simulink model "FOC_2020b"  (R2021a)
settings: Solver=ode23t  StartTime=0.0  StopTime=0.1  RelTol=1e-3  AbsTol=1e-3  EnableMultiTasking=on
values from neighbouring files (symbols this model uses):
  f_c = 10000    [FOC_params.m]
  Kpd = Ld*2*pi*BW    (= 0.0753982236862)    [FOC_params.m]
  Kpn = Kpq/(Lq*d*K)    (= 1.22461076833)    [FOC_params.m]
  Kpq = Lq*2*pi*BW    (= 0.125663706144)    [FOC_params.m]
  Kr = 270    [FOC_params.m]
  Ld = 0.00003    (= 3e-05)    [FOC_params.m]
  Lq = 0.00005    (= 5e-05)    [FOC_params.m]
  np = 5    [FOC_params.m]
  PERIOD = 3750    [FOC_params.m]
  psiPM = 0.007    [FOC_params.m]
  R = 0.023    [FOC_params.m]
  T_dead = 2.0e-6    (= 2e-06)    [FOC_params.m]
  Tnd = Ld/R    (= 0.00130434782609)    [FOC_params.m]
  Tnn = d^2*Lq/Kpq    (= 0.039788735773)    [FOC_params.m]
  Tnq = Lq/R    (= 0.00217391304348)    [FOC_params.m]
  u_dc = 12    [FOC_params.m]
libraries: nesl_utility x23, ee_lib x22, fl_lib x22, pid_lib x3, simulink x3, cstblocks x2, spsAlphaBetaZerotodq0Lib x1, spsabctoAlphaBetaZeroLib x1, spsdq0toAlphaBetaZeroLib x1, spsTriangleGeneratorLib x1
(part 2 of 2)

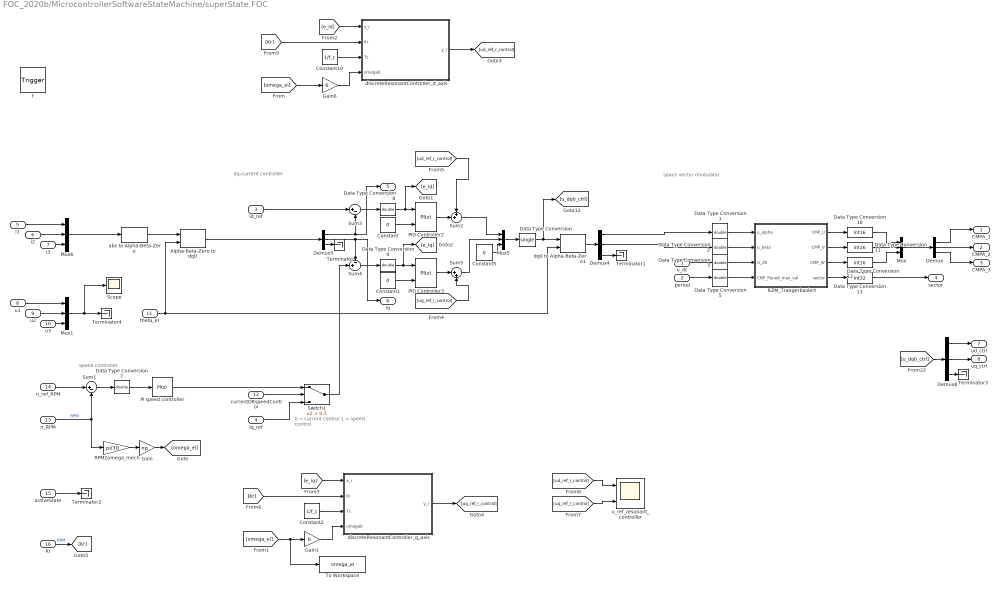
== system FOC_2020b/MicrocontrollerSoftwareStateMachine/superState.FOC ==
  note: speed controller
  note: space vector modulator
  note: dq-current controller
  note: 0 = current control
      | 1 = speed control
  u_dc : Inport  OutDataTypeStr=single  PortDimensions=1
  period : Inport  Port=2  OutDataTypeStr=uint16  PortDimensions=1
  id_ref : Inport  Port=3  OutDataTypeStr=single  PortDimensions=1
  iq_ref : Inport  Port=4  OutDataTypeStr=single  PortDimensions=1
  i1 : Inport  Port=5  OutDataTypeStr=single  PortDimensions=1
  i2 : Inport  Port=6  OutDataTypeStr=single  PortDimensions=1
  i3 : Inport  Port=7  OutDataTypeStr=single  PortDimensions=1
  u1 : Inport  Port=8  OutDataTypeStr=single  PortDimensions=1
  u2 : Inport  Port=9  OutDataTypeStr=single  PortDimensions=1
  u3 : Inport  Port=10  OutDataTypeStr=single  PortDimensions=1
  theta_el : Inport  Port=11  OutDataTypeStr=single  PortDimensions=1
  currentORspeedControl : Inport  Port=12  OutDataTypeStr=boolean  PortDimensions=1
  n_RPM : Inport  Port=13  OutDataTypeStr=single  PortDimensions=1
  n_ref_RPM : Inport  Port=14  OutDataTypeStr=single  PortDimensions=1
  activeState : Inport  Port=15  OutDataTypeStr=uint8  PortDimensions=1
  Kr : Inport  Port=16  OutDataTypeStr=single  PortDimensions=1
  f : TriggerPort  TriggerType=function-call  VariantControl=(inherit)
      settings: CopyFcn=Stateflow.SLINSF.SimulinkMan.removeBlockPreDeleteFcn  PreDeleteFcn=Stateflow.SLINSF.SimulinkMan.unsafePredeleteFcn
  Alpha-Beta-Zero to dq0 : spsAlphaBetaZerotodq0Lib/Alpha-Beta-Zero to dq0  Alignment=Aligned with phase A axis
      settings: SourceProductBaseCode=PS
  Constant : Constant  Value=0
  Constant1 : Constant  Value=0
  Constant10 : Constant  Value=1/f_c
  Constant2 : Constant  Value=1/f_c
  Constant5 : Constant  Value=0
  Data Type Conversion : DataTypeConversion  OutDataTypeStr=single
  Data Type Conversion{1..3,5,7..9} (7 alike) : DataTypeConversion  OutDataTypeStr=double
  Data Type Conversion10 : DataTypeConversion  OutDataTypeStr=int16
  Data Type Conversion11 : DataTypeConversion  OutDataTypeStr=int16
  Data Type Conversion12 : DataTypeConversion  OutDataTypeStr=int16
  Data Type Conversion13 : DataTypeConversion  OutDataTypeStr=int32
  Demux{,4..5,8} (4 alike) : Demux  Outputs=3
  Gain : Gain  Gain=np
  Gain1 : Gain  Gain=6
  Gain6 : Gain  Gain=6
  Mux{,1,5..6} (4 alike) : Mux  Inputs=3
  PI speed controller : pid_lib/PID Controller  Controller=PI  Form=Ideal  TimeDomain=Discrete-time  UseExternalTs=off  SampleTime=-1  IntegratorMethod=Forward Euler  FilterMethod=Forward Euler  ControllerParametersSource=internal  P=Kpn  I=1/Tnn  D=0  UseFilter=on  N=100  TunerSelectOption=Transfer Function Based (PID Tuner App)  InitialConditionSource=internal  InitialConditionForIntegrator=0  InitialConditionForFilter=0  DifferentiatorICPrevScaledInput=0  ExternalReset=none  TrackingMode=off  Kt=1  LimitOutput=on  SatLimitsSource=internal  UpperSaturationLimit=10  LowerSaturationLimit=-10  LinearizeAsGain=on  AntiWindupMode=clamping  Kb=1  POutMin=[]  POutMax=[]  IOutMin=[]  IOutMax=[]  DOutMin=[]  DOutMax=[]  NOutMin=[]  NOutMax=[]  SumOutMin=[]  SumOutMax=[]  SaturationOutMin=[]  SaturationOutMax=[]  PParamMin=[]  PParamMax=[]  IParamMin=[]  IParamMax=[]  DParamMin=[]  DParamMax=[]  NParamMin=[]  NParamMax=[]  KbParamMin=[]  KbParamMax=[]  KtParamMin=[]  KtParamMax=[]  KbOutMin=[]  KbOutMax=[]  KtOutMin=[]  KtOutMax=[]  IntegratorOutMin=[]  IntegratorOutMax=[]  FilterOutMin=[]  FilterOutMax=[]  SumI1OutMin=[]  SumI1OutMax=[]  SumI2OutMin=[]  SumI2OutMax=[]  SumI3OutMin=[]  SumI3OutMax=[]  SumI4OutMin=[]  SumI4OutMax=[]  SumDOutMin=[]  SumDOutMax=[]  DifferentiatorOutMin=[]  DifferentiatorOutMax=[]  FilterDiffOutCoefMin=[]  FilterDiffOutCoefMax=[]  ReciprocalOutMin=[]  ReciprocalOutMax=[]  SumDenOutMin=[]  SumDenOutMax=[]  SumNumOutMin=[]  SumNumOutMax=[]  DivideOutMin=[]  DivideOutMax=[]  UdiffTsProdOutMin=[]  UdiffTsProdOutMax=[]  NTsProdOutMin=[]  NTsProdOutMax=[]  UintegralTsProdOutMin=[]  UintegralTsProdOutMax=[]  UngainTsProdOutMin=[]  UngainTsProdOutMax=[]  IntegratorContinuousStateAttributes=''  IntegratorStateMustResolveToSignalObject=off  IntegratorRTWStateStorageClass=Auto  FilterContinuousStateAttributes=''  FilterStateMustResolveToSignalObject=off  FilterRTWStateStorageClass=Auto  ParallelPVariant=Passthrough  IdealPVariant=InternalParameters  IVariant=InternalParameters  DVariant=Disabled  IntegratorVariant=Discrete  SatVariant=Enabled  AWVariant=DiscClampingIdeal  PCopyVariant=InternalParamsIdeal  TRVariant=Disabled  FdbkBlocksVariant=Forward  IdealPFdbkVariant=Disabled  SatFdbkVariant=Disabled  DerivativeFilterVariant=Disabled  NVariant=Disabled  NCopyVariant=Disabled_SignalSpec  FilterICVariant=Disabled  IntegratorICVariant=InternalICs  ExternalResetVariant=Disabled  TRSumVariant=Passthrough  SumFdbkVariant=Disabled  SumVariant=Sum_PI  TsampFilterVariant=InternalTs  TsampNgainVariant=Passthrough  TsampIntegralVariant=Passthrough  ExternalSaturationOutDataTypeStr=Inherit: Same as second input
  PID Controller2 : pid_lib/PID Controller  Controller=PI  Form=Ideal  TimeDomain=Discrete-time  UseExternalTs=off  SampleTime=-1  IntegratorMethod=Forward Euler  FilterMethod=Forward Euler  ControllerParametersSource=internal  P=Kpd  I=1/Tnd  D=0  UseFilter=on  N=100  TunerSelectOption=Transfer Function Based (PID Tuner App)  InitialConditionSource=internal  InitialConditionForIntegrator=0  InitialConditionForFilter=0  DifferentiatorICPrevScaledInput=0  ExternalReset=rising  TrackingMode=off  Kt=1  LimitOutput=on  SatLimitsSource=internal  UpperSaturationLimit=12  LowerSaturationLimit=-12  LinearizeAsGain=on  AntiWindupMode=clamping  Kb=1  POutMin=[]  POutMax=[]  IOutMin=[]  IOutMax=[]  DOutMin=[]  DOutMax=[]  NOutMin=[]  NOutMax=[]  SumOutMin=[]  SumOutMax=[]  SaturationOutMin=[]  SaturationOutMax=[]  PParamMin=[]  PParamMax=[]  IParamMin=[]  IParamMax=[]  DParamMin=[]  DParamMax=[]  NParamMin=[]  NParamMax=[]  KbParamMin=[]  KbParamMax=[]  KtParamMin=[]  KtParamMax=[]  KbOutMin=[]  KbOutMax=[]  KtOutMin=[]  KtOutMax=[]  IntegratorOutMin=[]  IntegratorOutMax=[]  FilterOutMin=[]  FilterOutMax=[]  SumI1OutMin=[]  SumI1OutMax=[]  SumI2OutMin=[]  SumI2OutMax=[]  SumI3OutMin=[]  SumI3OutMax=[]  SumI4OutMin=[]  SumI4OutMax=[]  SumDOutMin=[]  SumDOutMax=[]  DifferentiatorOutMin=[]  DifferentiatorOutMax=[]  FilterDiffOutCoefMin=[]  FilterDiffOutCoefMax=[]  ReciprocalOutMin=[]  ReciprocalOutMax=[]  SumDenOutMin=[]  SumDenOutMax=[]  SumNumOutMin=[]  SumNumOutMax=[]  DivideOutMin=[]  DivideOutMax=[]  UdiffTsProdOutMin=[]  UdiffTsProdOutMax=[]  NTsProdOutMin=[]  NTsProdOutMax=[]  UintegralTsProdOutMin=[]  UintegralTsProdOutMax=[]  UngainTsProdOutMin=[]  UngainTsProdOutMax=[]  IntegratorContinuousStateAttributes=''  IntegratorStateMustResolveToSignalObject=off  IntegratorRTWStateStorageClass=Auto  FilterContinuousStateAttributes=''  FilterStateMustResolveToSignalObject=off  FilterRTWStateStorageClass=Auto  ParallelPVariant=Passthrough  IdealPVariant=InternalParameters  IVariant=InternalParameters  DVariant=Disabled  IntegratorVariant=Discrete  SatVariant=Enabled  AWVariant=DiscClampingIdeal  PCopyVariant=InternalParamsIdeal  TRVariant=Disabled  FdbkBlocksVariant=Forward  IdealPFdbkVariant=Disabled  SatFdbkVariant=Disabled  DerivativeFilterVariant=Disabled  NVariant=Disabled  NCopyVariant=Disabled_SignalSpec  FilterICVariant=Disabled  IntegratorICVariant=InternalICs  ExternalResetVariant=ExternalReset  TRSumVariant=Passthrough  SumFdbkVariant=Disabled  SumVariant=Sum_PI  TsampFilterVariant=InternalTs  TsampNgainVariant=Passthrough  TsampIntegralVariant=Passthrough  ExternalSaturationOutDataTypeStr=Inherit: Same as second input
  PID Controller3 : pid_lib/PID Controller  Controller=PI  Form=Ideal  TimeDomain=Discrete-time  UseExternalTs=off  SampleTime=-1  IntegratorMethod=Forward Euler  FilterMethod=Forward Euler  ControllerParametersSource=internal  P=Kpq  I=1/Tnq  D=0  UseFilter=on  N=100  TunerSelectOption=Transfer Function Based (PID Tuner App)  InitialConditionSource=internal  InitialConditionForIntegrator=0  InitialConditionForFilter=0  DifferentiatorICPrevScaledInput=0  ExternalReset=rising  TrackingMode=off  Kt=1  LimitOutput=on  SatLimitsSource=internal  UpperSaturationLimit=12  LowerSaturationLimit=-12  LinearizeAsGain=on  AntiWindupMode=clamping  Kb=1  POutMin=[]  POutMax=[]  IOutMin=[]  IOutMax=[]  DOutMin=[]  DOutMax=[]  NOutMin=[]  NOutMax=[]  SumOutMin=[]  SumOutMax=[]  SaturationOutMin=[]  SaturationOutMax=[]  PParamMin=[]  PParamMax=[]  IParamMin=[]  IParamMax=[]  DParamMin=[]  DParamMax=[]  NParamMin=[]  NParamMax=[]  KbParamMin=[]  KbParamMax=[]  KtParamMin=[]  KtParamMax=[]  KbOutMin=[]  KbOutMax=[]  KtOutMin=[]  KtOutMax=[]  IntegratorOutMin=[]  IntegratorOutMax=[]  FilterOutMin=[]  FilterOutMax=[]  SumI1OutMin=[]  SumI1OutMax=[]  SumI2OutMin=[]  SumI2OutMax=[]  SumI3OutMin=[]  SumI3OutMax=[]  SumI4OutMin=[]  SumI4OutMax=[]  SumDOutMin=[]  SumDOutMax=[]  DifferentiatorOutMin=[]  DifferentiatorOutMax=[]  FilterDiffOutCoefMin=[]  FilterDiffOutCoefMax=[]  ReciprocalOutMin=[]  ReciprocalOutMax=[]  SumDenOutMin=[]  SumDenOutMax=[]  SumNumOutMin=[]  SumNumOutMax=[]  DivideOutMin=[]  DivideOutMax=[]  UdiffTsProdOutMin=[]  UdiffTsProdOutMax=[]  NTsProdOutMin=[]  NTsProdOutMax=[]  UintegralTsProdOutMin=[]  UintegralTsProdOutMax=[]  UngainTsProdOutMin=[]  UngainTsProdOutMax=[]  IntegratorContinuousStateAttributes=''  IntegratorStateMustResolveToSignalObject=off  IntegratorRTWStateStorageClass=Auto  FilterContinuousStateAttributes=''  FilterStateMustResolveToSignalObject=off  FilterRTWStateStorageClass=Auto  ParallelPVariant=Passthrough  IdealPVariant=InternalParameters  IVariant=InternalParameters  DVariant=Disabled  IntegratorVariant=Discrete  SatVariant=Enabled  AWVariant=DiscClampingIdeal  PCopyVariant=InternalParamsIdeal  TRVariant=Disabled  FdbkBlocksVariant=Forward  IdealPFdbkVariant=Disabled  SatFdbkVariant=Disabled  DerivativeFilterVariant=Disabled  NVariant=Disabled  NCopyVariant=Disabled_SignalSpec  FilterICVariant=Disabled  IntegratorICVariant=InternalICs  ExternalResetVariant=ExternalReset  TRSumVariant=Passthrough  SumFdbkVariant=Disabled  SumVariant=Sum_PI  TsampFilterVariant=InternalTs  TsampNgainVariant=Passthrough  TsampIntegralVariant=Passthrough  ExternalSaturationOutDataTypeStr=Inherit: Same as second input
  RPM2omega_mech : Gain  Gain=pi/30
  RZM_Traegerbasiert : MATLAB Function  TreatAsAtomicUnit=on
  Scope : Scope
  Sum1 : Sum  Inputs=|+-
  Sum2 : Sum  Inputs=++|
  Sum3 : Sum  Inputs=|+-
  Sum4 : Sum  Inputs=-+|
  Sum5 : Sum  Inputs=|++
  Switch1 : Switch  Criteria=u2 > Threshold  Threshold=0.5
  Terminator{,1..4} (5 alike) : Terminator
  To Workspace : ToWorkspace  VariableName=omega_el  SaveFormat=Timeseries  SampleTime=-1
  abc to Alpha-Beta-Zero : spsabctoAlphaBetaZeroLib/abc to Alpha-Beta-Zero
      settings: SourceProductBaseCode=PS
  discreteResonantController_d_axis : Subsystem
  discreteResonantController_q_axis : Subsystem
  dq0 to Alpha-Beta-Zero1 : spsdq0toAlphaBetaZeroLib/dq0 to Alpha-Beta-Zero  Alignment=Aligned with phase A axis
      settings: SourceProductBaseCode=PS
  u_ref_resonant_controller : Scope  NumInputPorts=2
  CMPA_1 : Outport  OutDataTypeStr=int16  PortDimensions=1  VectorParamsAs1DForOutWhenUnconnected=off
  CMPA_2 : Outport  Port=2  OutDataTypeStr=int16  PortDimensions=1  VectorParamsAs1DForOutWhenUnconnected=off
  CMPA_3 : Outport  Port=3  OutDataTypeStr=int16  PortDimensions=1  VectorParamsAs1DForOutWhenUnconnected=off
  sector : Outport  Port=4  OutDataTypeStr=int32  PortDimensions=1  VectorParamsAs1DForOutWhenUnconnected=off
  id : Outport  Port=5  OutDataTypeStr=single  PortDimensions=1  VectorParamsAs1DForOutWhenUnconnected=off
  iq : Outport  Port=6  OutDataTypeStr=single  PortDimensions=1  VectorParamsAs1DForOutWhenUnconnected=off
  ud_ctrl : Outport  Port=7  OutDataTypeStr=single  PortDimensions=1  VectorParamsAs1DForOutWhenUnconnected=off
  uq_ctrl : Outport  Port=8  OutDataTypeStr=single  PortDimensions=1  VectorParamsAs1DForOutWhenUnconnected=off
  wires:
  i2/1 -> Mux6/2
  Demux4/3 -> Terminator1/1
  RZM_Traegerbasiert/1(CMP_U) -> Data Type Conversion10/1
  Constant5/1 -> Mux5/3
  dq0 to Alpha-Beta-Zero1/1 -> Demux4/1
  Demux5/2 -> iq/1, Sum4/1
  Demux5/3 -> Terminator/1
  Sum3/1 -> Data Type Conversion8/1
  Data Type Conversion1/1 -> RZM_Traegerbasiert/1(u_alpha)
  i3/1 -> Mux6/3
  Demux5/1 -> id/1, Sum3/2
  Data Type Conversion2/1 -> RZM_Traegerbasiert/2(u_beta)
  Alpha-Beta-Zero to dq0/1 -> Demux5/1
  Mux5/1 -> Data Type Conversion/1
  RZM_Traegerbasiert/3(CMP_W) -> Data Type Conversion12/1
  Switch1/1 -> Sum4/2
  Sum4/1 -> Data Type Conversion9/1
  u_dc/1 -> Data Type Conversion3/1
  RZM_Traegerbasiert/2(CMP_V) -> Data Type Conversion11/1
  RZM_Traegerbasiert/4(sector) -> Data Type Conversion13/1
  Data Type Conversion3/1 -> RZM_Traegerbasiert/3(U_ZK)
  id_ref/1 -> Sum3/1
  Data Type Conversion5/1 -> RZM_Traegerbasiert/4(CMP_Period_max_val)
  Data Type Conversion/1 -> [u_dq0_ctrl], dq0 to Alpha-Beta-Zero1/1
  Data Type Conversion8/1 -> [e_id], PID Controller2/1
  Data Type Conversion9/1 -> [e_iq], PID Controller3/1
  Demux4/1 -> Data Type Conversion1/1
  Demux4/2 -> Data Type Conversion2/1
  period/1 -> Data Type Conversion5/1
  Data Type Conversion11/1 -> Mux/2
  Data Type Conversion10/1 -> Mux/1
  Data Type Conversion12/1 -> Mux/3
  Mux/1 -> Demux/1
  Data Type Conversion13/1 -> sector/1
  i1/1 -> Mux6/1
  u1/1 -> Mux1/1
  u2/1 -> Mux1/2
  u3/1 -> Mux1/3
  Mux6/1 -> abc to Alpha-Beta-Zero/1
  abc to Alpha-Beta-Zero/1 -> Alpha-Beta-Zero to dq0/1
  Mux1/1 -> Scope/1, Terminator4/1
  theta_el/1 -> dq0 to Alpha-Beta-Zero1/2, Alpha-Beta-Zero to dq0/2
  iq_ref/1 -> Switch1/3
  currentORspeedControl/1 -> Switch1/2
  Data Type Conversion7/1 -> PI speed controller/1
  PI speed controller/1 -> Switch1/1
  Sum1/1 -> Data Type Conversion7/1
  n_ref_RPM/1 -> Sum1/1
  Constant1/1 -> PID Controller3/2
  Constant/1 -> PID Controller2/2
  activeState/1 -> Terminator2/1
  [u_dq0_ctrl] -> Demux8/1
  Demux8/3 -> Terminator3/1
  Demux8/2 -> uq_ctrl/1
  Demux8/1 -> ud_ctrl/1
  Demux/1 -> CMPA_1/1
  Demux/3 -> CMPA_3/1
  Demux/2 -> CMPA_2/1
  PID Controller2/1 -> Sum2/2
  PID Controller3/1 -> Sum5/1
  n_RPM/1 -> RPM2omega_mech/1, Sum1/2  "RPM"
  Gain6/1 -> discreteResonantController_d_axis/4(omega0)
  [Kr] -> discreteResonantController_d_axis/2(Kr)
  [omega_el] -> Gain6/1
  [e_id] -> discreteResonantController_d_axis/1(x_r)
  Constant10/1 -> discreteResonantController_d_axis/3(Ts)
  discreteResonantController_d_axis/1(y_r) -> [ud_ref_r_control]
  [omega_el] -> To Workspace/1, Gain1/1
  discreteResonantController_q_axis/1(y_r) -> [uq_ref_r_control]
  [e_iq] -> discreteResonantController_q_axis/1(x_r)
  Constant2/1 -> discreteResonantController_q_axis/3(Ts)
  Gain1/1 -> discreteResonantController_q_axis/4(omega0)
  Sum2/1 -> Mux5/1
  Sum5/1 -> Mux5/2
  RPM2omega_mech/1 -> Gain/1
  Gain/1 -> [omega_el]
  [uq_ref_r_control] -> Sum5/2
  [ud_ref_r_control] -> Sum2/1
  [Kr] -> discreteResonantController_q_axis/2(Kr)
  Kr/1 -> [Kr]  "RPM"
  [uq_ref_r_control] -> u_ref_resonant_controller/2
  [ud_ref_r_control] -> u_ref_resonant_controller/1

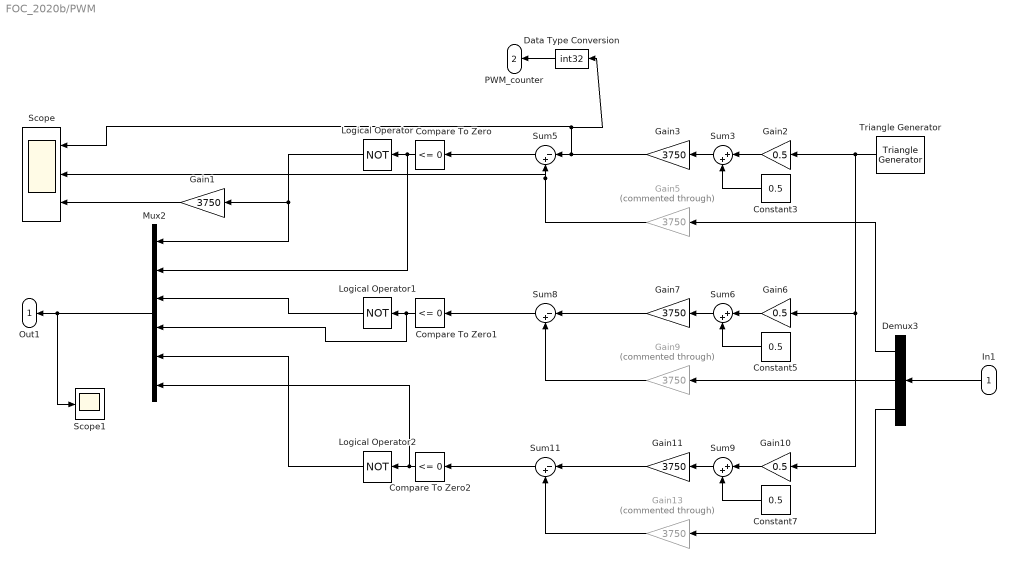
== system FOC_2020b/PWM ==
  In1 : Inport
  Compare To Zero : simulink/Logic and Bit Operations/Compare To Zero  relop=<=  OutDataTypeStr=boolean
  Compare To Zero1 : simulink/Logic and Bit Operations/Compare To Zero  relop=<=  OutDataTypeStr=boolean
  Compare To Zero2 : simulink/Logic and Bit Operations/Compare To Zero  relop=<=  OutDataTypeStr=boolean
  Constant3 : Constant  Value=0.5
  Constant5 : Constant  Value=0.5
  Constant7 : Constant  Value=0.5
  Data Type Conversion : DataTypeConversion  OutDataTypeStr=int32
  Demux3 : Demux  Outputs=3
  Gain{1,3,7,11} (4 alike) : Gain  Gain=3750  ParamDataTypeStr=single
  Gain10 : Gain  Gain=0.5
  Gain13 : Gain  Commented=through  Gain=3750  ParamDataTypeStr=single
  Gain2 : Gain  Gain=0.5
  Gain5 : Gain  Commented=through  Gain=3750  ParamDataTypeStr=single
  Gain6 : Gain  Gain=0.5
  Gain9 : Gain  Commented=through  Gain=3750  ParamDataTypeStr=single
  Logical Operator : Logic  Operator=NOT  AllPortsSameDT=off  OutDataTypeStr=boolean
  Logical Operator1 : Logic  Operator=NOT  AllPortsSameDT=off  OutDataTypeStr=boolean
  Logical Operator2 : Logic  Operator=NOT  AllPortsSameDT=off  OutDataTypeStr=boolean
  Mux2 : Mux  Inputs=6
  Scope : Scope  NumInputPorts=3
  Scope1 : Scope
  Sum11 : Sum  Inputs=|-+
  Sum3 : Sum  Inputs=|++
  Sum5 : Sum  Inputs=|-+
  Sum6 : Sum  Inputs=|++
  Sum8 : Sum  Inputs=|-+
  Sum9 : Sum  Inputs=|++
  Triangle Generator : spsTriangleGeneratorLib/Triangle Generator  Freq=20000  Phase=0  Ts=0
  Out1 : Outport  VectorParamsAs1DForOutWhenUnconnected=off
  PWM_counter : Outport  Port=2  VectorParamsAs1DForOutWhenUnconnected=off
  wires:
  Demux3/3 -> Gain13/1
  Logical Operator2/1 -> Mux2/5
  Logical Operator1/1 -> Mux2/3
  Mux2/1 -> Scope1/1, Out1/1
  Compare To Zero2/1 -> Mux2/6, Logical Operator2/1
  Gain10/1 -> Sum9/1
  Sum8/1 -> Compare To Zero1/1
  Gain6/1 -> Sum6/1
  Sum9/1 -> Gain11/1
  Triangle Generator/1 -> Gain10/1, Gain6/1, Gain2/1
  Sum6/1 -> Gain7/1
  Demux3/2 -> Gain9/1
  Compare To Zero1/1 -> Mux2/4, Logical Operator1/1
  Constant5/1 -> Sum6/2
  Constant7/1 -> Sum9/2
  Sum11/1 -> Compare To Zero2/1
  Sum3/1 -> Gain3/1
  Constant3/1 -> Sum3/2
  Demux3/1 -> Gain5/1
  Sum5/1 -> Compare To Zero/1
  Gain2/1 -> Sum3/1
  In1/1 -> Demux3/1
  Gain5/1 -> Scope/2, Sum5/2
  Gain9/1 -> Sum8/2
  Gain13/1 -> Sum11/2
  Gain3/1 -> Data Type Conversion/1, Scope/1, Sum5/1
  Gain7/1 -> Sum8/1
  Gain11/1 -> Sum11/1
  Logical Operator/1 -> Gain1/1, Mux2/1
  Compare To Zero/1 -> Mux2/2, Logical Operator/1
  Gain1/1 -> Scope/3
  Data Type Conversion/1 -> PWM_counter/1

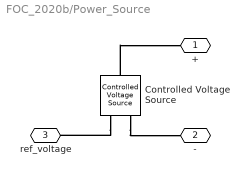
== system FOC_2020b/Power_Source ==
  Controlled Voltage Source : fl_lib/Electrical/Electrical Sources/Controlled Voltage Source
  + : PMIOPort  Side=Right
  - : PMIOPort  Port=2  Side=Right
  ref_voltage : PMIOPort  Port=3  Side=Left
  connections:
  Controlled Voltage Source/LConn1 -- +/RConn1
  Controlled Voltage Source/RConn2 -- -/RConn1
  Controlled Voltage Source/RConn1 -- ref_voltage/RConn1

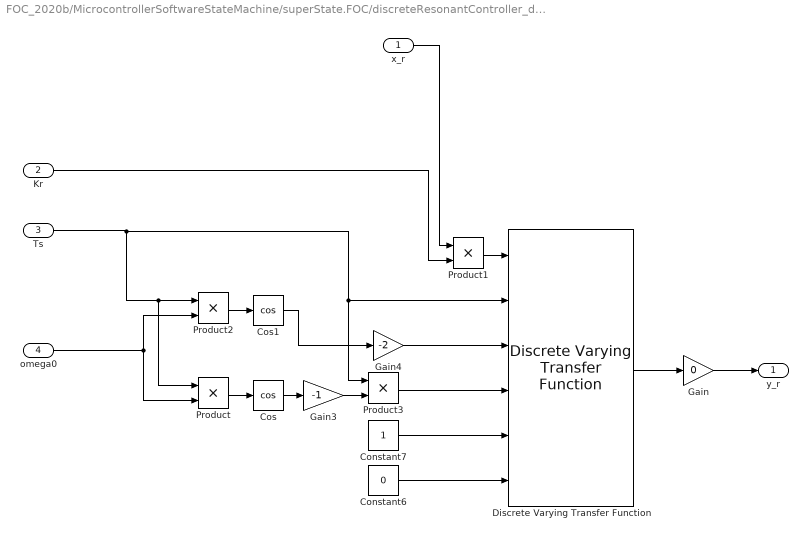
== system FOC_2020b/MicrocontrollerSoftwareStateMachine/superState.FOC/discreteResonantController_d_axis ==
  x_r : Inport
  Kr : Inport  Port=2
  Ts : Inport  Port=3
  omega0 : Inport  Port=4
  Constant6 : Constant  Value=0
  Constant7 : Constant
  Cos : Trigonometry  Operator=cos
  Cos1 : Trigonometry  Operator=cos
  Discrete Varying Transfer Function : cstblocks/Linear Parameter Varying/Discrete Varying Transfer Function  N=2  Ts=-1
      settings: SourceProductBaseCode=CT
  Gain : Gain  Gain=0
  Gain3 : Gain  Gain=-1
  Gain4 : Gain  Gain=-2
  Product{,1..3} (4 alike) : Product
  y_r : Outport  VectorParamsAs1DForOutWhenUnconnected=off
  wires:
  Constant6/1 -> Discrete Varying Transfer Function/6
  Ts/1 -> Discrete Varying Transfer Function/2, Product3/1, Product/1, Product2/1
  Cos/1 -> Gain3/1
  Cos1/1 -> Gain4/1
  Product2/1 -> Cos1/1
  Gain4/1 -> Discrete Varying Transfer Function/3
  Constant7/1 -> Discrete Varying Transfer Function/5
  Product/1 -> Cos/1
  Product1/1 -> Discrete Varying Transfer Function/1
  Gain3/1 -> Product3/2
  x_r/1 -> Product1/1
  Product3/1 -> Discrete Varying Transfer Function/4
  omega0/1 -> Product/2, Product2/2
  Discrete Varying Transfer Function/1 -> Gain/1
  Kr/1 -> Product1/2
  Gain/1 -> y_r/1

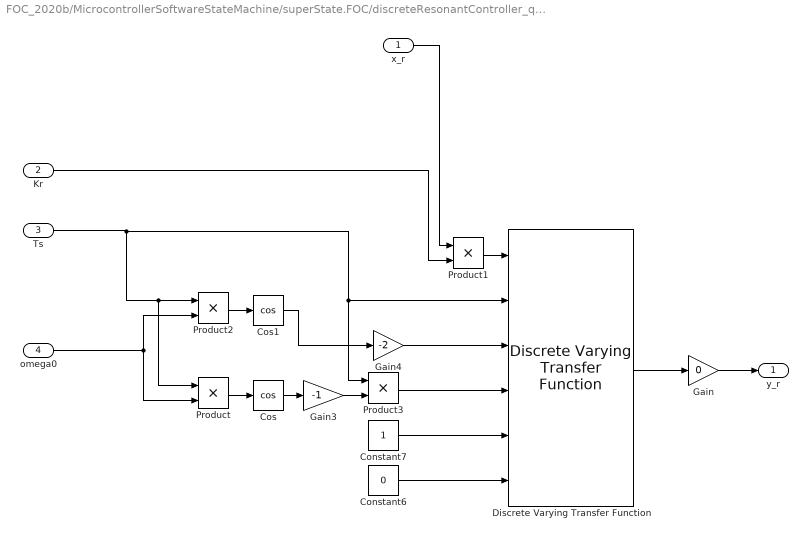
== system FOC_2020b/MicrocontrollerSoftwareStateMachine/superState.FOC/discreteResonantController_q_axis ==
  x_r : Inport
  Kr : Inport  Port=2
  Ts : Inport  Port=3
  omega0 : Inport  Port=4
  Constant6 : Constant  Value=0
  Constant7 : Constant
  Cos : Trigonometry  Operator=cos
  Cos1 : Trigonometry  Operator=cos
  Discrete Varying Transfer Function : cstblocks/Linear Parameter Varying/Discrete Varying Transfer Function  N=2  Ts=-1
      settings: SourceProductBaseCode=CT
  Gain : Gain  Gain=0
  Gain3 : Gain  Gain=-1
  Gain4 : Gain  Gain=-2
  Product{,1..3} (4 alike) : Product
  y_r : Outport  VectorParamsAs1DForOutWhenUnconnected=off
  wires:
  Constant6/1 -> Discrete Varying Transfer Function/6
  Ts/1 -> Discrete Varying Transfer Function/2, Product3/1, Product/1, Product2/1
  Cos/1 -> Gain3/1
  Cos1/1 -> Gain4/1
  Product2/1 -> Cos1/1
  Gain4/1 -> Discrete Varying Transfer Function/3
  Constant7/1 -> Discrete Varying Transfer Function/5
  Product/1 -> Cos/1
  Product1/1 -> Discrete Varying Transfer Function/1
  Gain3/1 -> Product3/2
  x_r/1 -> Product1/1
  Product3/1 -> Discrete Varying Transfer Function/4
  omega0/1 -> Product/2, Product2/2
  Discrete Varying Transfer Function/1 -> Gain/1
  Kr/1 -> Product1/2
  Gain/1 -> y_r/1

== matlab function FOC_2020b/3ph_Inverter/12bit ADC ==
  data: u input; y output
function y = fcn(u)
%#codegen

y = u*4095/3.3;

== matlab function FOC_2020b/3ph_Inverter/12bit ADC1 ==
  data: u input; y output
function y = fcn(u)
%#codegen

y = u*4095/3.3;

== matlab function FOC_2020b/3ph_Inverter/12bit ADC2 ==
  data: u input; y output
function y = fcn(u)
%#codegen

y = u*4095/3.3;

== stateflow chart FOC_2020b/MicrocontrollerSoftwareStateMachine ==
  settings: updateMethod=DISCRETE  sampleTime=1/f_c
  state superState
    state Init     %state 10
      entry:
      activeState = 10;
      CMPA_1 = 0;
      CMPA_2 = 0;
      CMPA_3 = 0;
      during:
      exit:
    state FieldOrientedControl     %state 20
      entry:
      activeState = 20;
      during:
      [CMPA_1,CMPA_2,CMPA_3,sector,id,iq,ud_ctrl,uq_ctrl] = FOC(u_dc,PERIOD,id_ref,iq_ref,i1,i2,i3,u1,u2,u3,theta_el,currentORspeedControl, n_RPM, n_ref_RPM, activeState,Kr)
    state [CMPA_1,CMPA_2,CMPA_3,sector,id,iq,ud_ctrl,uq_ctrl] = FOC(u_dc,period,id_ref,iq_ref,i1,i2,i3,u1,u2,u3,theta_el,currentORspeedControl,n_RPM,n_ref_RPM,activeState,Kr) [function]
    superState -> Init     %state 10 : [RESET == 1]
    (default) -> Init     %state 10
    Init     %state 10 -> FieldOrientedControl     %state 20 : [NEXT == 1]
  data: u_dc function_input single size=1; period function_input uint16 size=1; id_ref function_input single size=1; iq_ref function_input single size=1; i1 function_input single size=1; i2 function_input single size=1; i3 function_input single size=1; u1 function_input single size=1; u2 function_input single size=1; u3 function_input single size=1; theta_el function_input single size=1; CMPA_1 function_output int16 size=1; CMPA_2 function_output int16 size=1; CMPA_3 function_output int16 size=1; sector function_output int32 size=1; currentORspeedControl function_input boolean size=1; n_RPM function_input single size=1; n_ref_RPM function_input single size=1; activeState function_input uint8 size=1; id function_output single size=1; iq function_output single size=1; ud_ctrl function_output single size=1; uq_ctrl function_output single size=1; Kr function_input single size=1; activeState output uint8 size=1 =uint8(0); RESET input boolean size=1; NEXT input boolean size=1; u_dc input single size=1; PERIOD input uint16 size=1; id_ref input single size=1; iq_ref input single size=1; i1 input single size=1; i2 input single size=1; i3 input single size=1; theta_el input single size=1; CMPA_1 output int16 size=1 =int16(0); CMPA_2 output int16 size=1 =int16(0); CMPA_3 output int16 size=1 =int16(0); sector output int32 size=1 =int32(0); counter local uint32 size=1 =uint32(0); u1 input single size=1; u2 input single size=1; u3 input single size=1; Rs input single size=1; Ls input single size=1; psiPM input single size=1; currentORspeedControl input boolean size=1; n_ref_RPM input single size=1; n_RPM input single size=1; id output single size=1 =single(0); iq output single size=1 =single(0); ud_ctrl output; uq_ctrl output; Kr input

== matlab function FOC_2020b/MicrocontrollerSoftwareStateMachine/superState.FOC/RZM_Traegerbasiert ==
  data: u_alpha input; u_beta input; U_ZK input; CMP_U output; CMP_Period_max_val input; CMP_V output; CMP_W output; sector output
function [CMP_U, CMP_V, CMP_W, sector] = fcn(u_alpha, u_beta, U_ZK, CMP_Period_max_val)
%#codegen

a_U_on=0;
a_V_on=0;
a_W_on=0;
CMP_U=0;
CMP_V=0;
CMP_W=0;

 %%__%%__%%__%%__%%__%%__%%__%%__%%__%%__%%__%%__%%__%%__%%__%%__%%__%%__%%_
    %%Trägerbasierte Raumzeigermodulation%%
    %%Eingänge:
    %U_ZK       -- Zwischenkreisspannung
    %u_alpha    -- alphakomponente des Sollspannungsraumzeigers
    %u_beta     -- betakomponente des Sollspannungsraumzeigers
    %CMP_Period_max_val  -- maximalwert des Dreiecks/Sägezahnzählers zum Gewichten der Aussteuergrade
    %%Ausgänge:
    %CMP_U        -- Vergleichswert U
    %CMP_V        -- Vergleichswert V
    %CMP_W        -- Vergleichswert W
    %sector       -- Ausgabe des Sektors des Spannungszeigers
    
    
    %Berechnung von a, b, c nach Quang Dittrich S24
    
    a = abs(u_alpha) + 0.5774*abs(u_beta);
    b = abs(u_alpha) - 0.5774*abs(u_beta);
    c = 1.1547*abs(u_beta);
    
    
    %Sektor und Quadranten nach Quang Dittrich S32
    if(u_beta < 0)
        if (u_alpha <0)
            quadrant=3;
            if(b < 0)
                sector = 5;
            else
                sector = 4;
            end
        else
            quadrant=4;
            if(b < 0)
                sector = 5;
            else
                sector = 6;
            end
        end
        
    else
        if (u_alpha <0)
            quadrant=2;
            if(b < 0)
                sector = 2;
            else
                sector = 3;
            end
        else
            quadrant=1;
            if(b < 0)
                sector = 2;
            else
                sector = 1;
            end
        end
    end
    
    sector = sector;
    
    %%Modulationsfunktionen für Phasen U,V,W
    %%Erzeugung der Aussteuergrade für die Halbbrücken
    %%--> Erzeugung einer "regulary Sampled SVM" erfolgt anschließend durch Abtastung
    %%mit Dreieckszählern in Hardware.
    
    if (sector == 1)
        
        u1 = b/(0.66667*U_ZK);
        u2 = c/(0.66667*U_ZK);
        
        a_U_on = 0.5 + u1*0.5 + u2*0.5;
        a_V_on = 0.5 - u1*0.5 + u2*0.5;
        a_W_on = 0.5 - u1*0.5 - u2*0.5;
    end
    
    
    if ((sector == 2) && (quadrant == 1))
        
        u1 = a/(0.66667*U_ZK);
        u2 = (-abs(u_alpha) + 0.5774*abs(u_beta))/(0.66667*U_ZK);
        
        a_U_on = 0.5 + u1*0.5 - u2*0.5;
        a_V_on = 0.5 + u1*0.5 + u2*0.5;
        a_W_on = 0.5 - u1*0.5 - u2*0.5;
    end
    
    
    if ((sector == 2) && (quadrant == 2))
        
        u1 = (-abs(u_alpha) + 0.5774*abs(u_beta))/(0.66667*U_ZK);
        u2 = a/(0.66667*U_ZK);
        
        a_U_on = 0.5 + u1*0.5 - u2*0.5;
        a_V_on = 0.5 + u1*0.5 + u2*0.5;
        a_W_on = 0.5 - u1*0.5 - u2*0.5;
    end
    
    
    if (sector == 3)
        
        u1 = c/(0.66667*U_ZK);
        u2 = b/(0.66667*U_ZK);
        
        a_U_on=  0.5 - u1*0.5 - u2*0.5;
        a_V_on = 0.5 + u1*0.5 + u2*0.5;
        a_W_on = 0.5 - u1*0.5 + u2*0.5;
    end
    
    if (sector == 4)
        
        u1 = b/(0.66667*U_ZK);
        u2 = c/(0.66667*U_ZK);
        
        a_U_on = 0.5 - u1*0.5 - u2*0.5;
        a_V_on = 0.5 + u1*0.5 - u2*0.5;
        a_W_on = 0.5 + u1*0.5 + u2*0.5;
    end
    
    
    if ((sector == 5) && (quadrant == 3))
        
        u1 = a/(0.66667*U_ZK);
        u2 = (-abs(u_alpha) + 0.5774*abs(u_beta))/(0.66667*U_ZK);
        
        a_U_on = 0.5 - u1*0.5 + u2*0.5;
        a_V_on = 0.5 - u1*0.5 - u2*0.5;
        a_W_on = 0.5 + u1*0.5 + u2*0.5;
    end
    
    
    if ((sector == 5) && (quadrant == 4))
        
        u1 =(-abs(u_alpha) + 0.5774*abs(u_beta))/(0.66667*U_ZK);
        u2 =  a/(0.66667*U_ZK);
        
        a_U_on = 0.5 - u1*0.5 + u2*0.5;
        a_V_on = 0.5 - u1*0.5 - u2*0.5;
        a_W_on = 0.5 + u1*0.5 + u2*0.5;
    end
    
    
    if (sector == 6)
        
        u1 = c/(0.66667*U_ZK);
        u2 = b/(0.66667*U_ZK);
        
        a_U_on = 0.5 + u1*0.5 + u2*0.5;
        a_V_on = 0.5 - u1*0.5 - u2*0.5;
        a_W_on = 0.5 + u1*0.5 - u2*0.5;
    end
    
    
    %%Aussteuergrade auf Zählregister normieren -> Comparewerte CMP
    CMP_U = a_U_on * CMP_Period_max_val;
    CMP_V = a_V_on * CMP_Period_max_val;
    CMP_W = a_W_on * CMP_Period_max_val;
    
    %%Begrenzung
    if (CMP_U > CMP_Period_max_val)
        CMP_U = CMP_Period_max_val;
    end
    if (CMP_U < 0)
        CMP_U = 0;
    end
    
    if (CMP_V > CMP_Period_max_val)
        CMP_V = CMP_Period_max_val;
    end
    if (CMP_V < 0)
        CMP_V = 0;
    end
    
    if (CMP_W > CMP_Period_max_val)
        CMP_W = CMP_Period_max_val;
    end
    if (CMP_W < 0)
        CMP_W = 0;
    end
    %%__%%__%%__%%__%%__%%__%%__%%__%%__%%__%%__%%__%%__%%__%%__%%__%%__%%__%%_
